simulink model "PEM_cell_validate_static"  (R2025b)
settings: Solver=ode23t  StartTime=0.0  StopTime=6895  RelTol=1e-3
values from neighbouring files (symbols this model uses):
  Active_Area = 17.64    [PV_PEM_direct_battery_active.m]    (also in PV_PEM_direct_battery_passive.m; PV_PEM_indirect_battery.m; PV_PEM_reconfigurable_battery.m; Sim_vs_meas_dynamic.m)
  Input_Time = T{:,5}    [Sim_vs_meas_dynamic.m]
  Input_Voltage = T{:,16}    [Sim_vs_meas_dynamic.m]
  Ra = 0.00177    [PV_PEM_direct_battery_active.m]    (also in PV_PEM_direct_battery_passive.m; PV_PEM_indirect_battery.m; PV_PEM_reconfigurable_battery.m; Sim_vs_meas_dynamic.m)
  Rc = 0.0005    [PV_PEM_direct_battery_active.m]    (also in PV_PEM_direct_battery_passive.m; PV_PEM_indirect_battery.m; PV_PEM_reconfigurable_battery.m; Sim_vs_meas_dynamic.m)
  Rint = 0.008673    [PV_PEM_direct_battery_active.m]    (also in PV_PEM_direct_battery_passive.m; PV_PEM_indirect_battery.m; PV_PEM_reconfigurable_battery.m; Sim_vs_meas_dynamic.m)
  Vint = 1.475841    [PV_PEM_direct_battery_active.m]    (also in PV_PEM_direct_battery_passive.m; PV_PEM_indirect_battery.m; PV_PEM_reconfigurable_battery.m; Sim_vs_meas_dynamic.m)
libraries: fl_lib x15, nesl_utility x9, simulink x6
settings Model: Creator=hanna  LastModifiedBy=hanna
settings DataIOCC: SignalLogging=off  StreamToWks=off  ReturnWorkspaceOutputs=off
settings DebuggingCC: SaveWithParameterizedLinksMsg=none

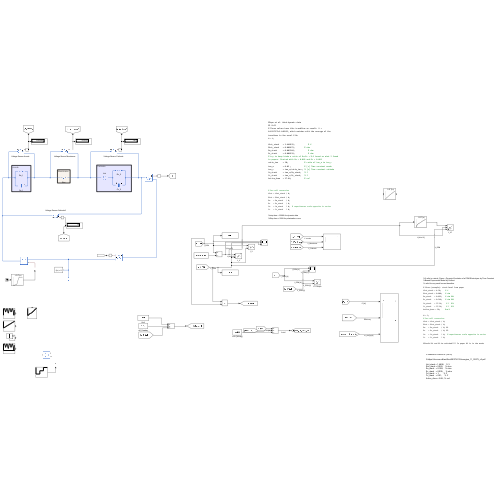
[thumbnail: Simulink's stored preview of the top-level diagram]
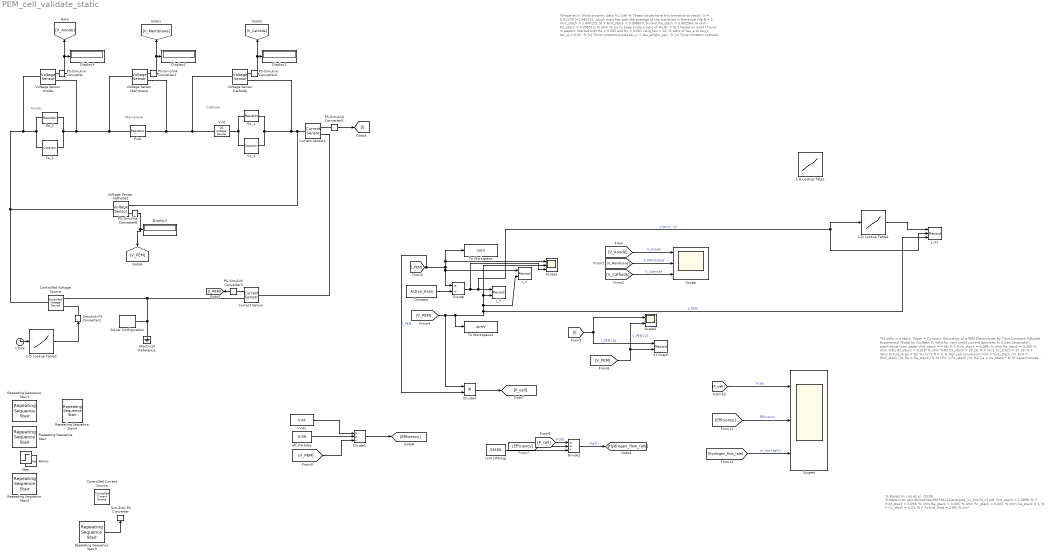
== system PEM_cell_validate_static ==
  note: %Pape et al. Wind dynamic data
      | %1 Cell
      | % These values have this trendline as result: V = 0.01175*I+1.440125, which matches with the average of the trendines in the excel file
      | N = 1;
      |
      | Vint_stack = 1.440155; % V
      | Rint_stack = 0.008673; % ohm
      | Ra_stack = 0.002564; % ohm
      | Rc_stack = 0.000513; % ohm
      | % try to keep kinda a ratio of Ra:Rc = %:1 based on what I found in papers. Started with Ra = 0.005 and Rc = 0.001
      | ratio_tau = 10; % ratio of tau_a to tau_c
      | tau_a = 0.05 ; % [s] Time constant anode
      | tau_c = tau_a/ratio_tau ; % [s] Time constant cathode
      | Ca_stack = tau_a/Ra_stack; % F
      | Cc_stack = tau_c/Rc_stack; % F
      | Active_Area = 17.64; % cm²
      |
      | % Per-cell conversion
      | Vint = Vint_stack / N;
      | Rint = Rint_stack / N;
      | Ra = Ra_stack / N;
      | Rc = Rc_stack / N;
      | Ca = Ca_stack * N; % capacitances scale opposite in series
      | Cc = Cc_stack * N;
      |
      | %stop time = 29988 for dynamic data
      | %Stop time = 5099 for polarisation curve
  note: % Based on Liso et al. (2018)
      | %https://vbn.aau.dk/ws/files/293736112/energies_11_03273_v2.pdf
      | Vint_stack = 1.4898; % V
      | Rint_stack = 0.093; % ohm
      | Ra_stack = 0.005; % ohm
      | Rc_stack = 0.005; % ohm
      | Ca_stack = 1; % F
      | Cc_stack = 0.01; % F
      | Active_Area = 2.89; % cm²
  note: %3 cells in a stack: Paper = Dynamic Emulation of a PEM Electrolyzer by Time Constant %Based Exponential Model by Guilbert
      | % valid for very small current densities
      |
      | % Given (example): stack-level from paper
      | Vint_stack = 4.38; % V
      | Rint_stack = 0.088; % ohm
      | Ra_stack = 0.035; % ohm %R1
      | Rc_stack = 0.318; % ohm %R2
      | Ca_stack = 37.26; % F %C1
      | Cc_stack = 37.26; % F %C2
      | Active_Area = 50; %cm^2
      |
      | N = 3;
      | % Per-cell conversion
      | Vint = Vint_stack / N;
      | Rint = Rint_stack / N;
      | Ra = Ra_stack / N; %1
      | Rc = Rc_stack / N; %2
      | Ca = Ca_stack * N; % capacitances scale opposite in series
      | Cc = Cc_stack * N;
      |
      | %Should R1 and R2 be switched???? In paper R2 is in the anode
  note: Cathode
  note: Anode
  note: Membrane
  1-D Lookup Table : Lookup_n-D  NumberOfTableDimensions=1  BreakpointsForDimension1=|  Table=|  InternalRulePriority=Speed  RndMeth=Simplest
      BreakpointsForDimension1=|
      | [0.0385
      | 0.0963
      | 0.1784
      | 0.3065
      | 0.4043
      | 0.6017
      | 0.8000
      | 0.9971
      | 1.1935
      | 1.3913
      | 1.5897
      | 1.7870
      | 1.9839 ]
      Table=|
      | [1.4682
      | 1.5069
      | 1.5423
      | 1.5870
      | 1.6183
      | 1.6780
      | 1.7357
      | 1.7924
      | 1.8478
      | 1.8992
      | 1.9511
      | 1.9983
      | 2.0476 ]
  1-D Lookup Table1 : Lookup_n-D  NumberOfTableDimensions=1  BreakpointsForDimension1=[0.002196, 0.005037, 0.010062, 0.020117, 0.030138, 0.040142, 0.060187, 0.080224, 0.100238, 0.150326, 0.200385, 0.250495, 0.297237, 0.347374, 0.397259, 0.447324, 0.497136, 0.597415, 0.697348, 0.79707, 0.99733, 1.097498, 1.197311, 1.297265, 1.397199, 1.497192, 1.597162, 1.696959, 1.79709, 1.896997, 1.997028]  Table=[1.320659, 1.36234, 1.375311, 1.392194, 1.403544, 1.412891, 1.429582, 1.444366, 1.456766, 1.485284, 1.509416, 1.531258, 1.548522, 1.565118, 1.580856, 1.596021, 1.60947, 1.636368, 1.660976, 1.686156, 1.734229, 1.758361, 1.782015, 1.806052, 1.829134, 1.853552, 1.875967, 1.899622, 1.924231, 1.948363, 1.971923]  InternalRulePriority=Speed  RndMeth=Simplest
  1-D Lookup Table2 : Lookup_n-D  NumberOfTableDimensions=1  BreakpointsForDimension1=Input_Time  Table=Input_Voltage  InternalRulePriority=Speed  RndMeth=Simplest
  Ca_1 : fl_lib/Electrical/Electrical Elements/Capacitor  c=Ca F  r=1e-6 Ohm  g=0 1/Ohm  i_specify=off  i_priority=None  i=0 A  i_nominal_specify=off  i_nominal_value=1  i_nominal_unit=A  v_specify=off  v_priority=None  v=0 V  v_nominal_specify=off  v_nominal_value=1  v_nominal_unit=V  vc_specify=off  vc_priority=High  vc=0 V  vc_nominal_specify=off  vc_nominal_value=1  vc_nominal_unit=V
  Cc_2 : fl_lib/Electrical/Electrical Elements/Capacitor  c=Cc F  r=1e-6 Ohm  g=0 1/Ohm  i_specify=off  i_priority=None  i=0 A  i_nominal_specify=off  i_nominal_value=1  i_nominal_unit=A  v_specify=off  v_priority=None  v=0 V  v_nominal_specify=off  v_nominal_value=1  v_nominal_unit=V  vc_specify=off  vc_priority=High  vc=0 V  vc_nominal_specify=off  vc_nominal_value=1  vc_nominal_unit=V
  Clock : Clock
  Constant : Constant  Value=Active_Area
  Controlled Current Source : fl_lib/Electrical/Electrical Sources/Controlled Current Source
  Controlled Voltage Source : fl_lib/Electrical/Electrical Sources/Controlled Voltage Source
  Current Sensor : fl_lib/Electrical/Electrical Sensors/Current Sensor
  Current Sensor1 : fl_lib/Electrical/Electrical Sensors/Current Sensor
  Display{1..4} (4 alike) : Display
  Divide : Product  Inputs=*/
  Divide1 : Product  Inputs=**/
  Divide2 : Product  Inputs=**/
  Divide4 : Product  Inputs=**
  Electrical Reference : fl_lib/Electrical/Electrical Elements/Electrical Reference
  I_V : Record  NumPorts=2.0  FileSettingsInternal="{\"entries\":[{\"content\":{\"excelSettings\":{\"content\":{},\"type\":\"Streamout.ExcelSettings\"},\"parquetSettings\":{\"content\":{},\"type\":\"Streamout.ParquetSettings\"}},\"type\":\"Streamout.FileSettingStorage\",\"uuid\":\"\"}],\"packageUris\":[\"http:\\/\\/schema.mathworks.com\\/mf0\\/streamout_blocks\\/R2020a\"],\"version\":\"1.0\"}"  FrameSettings=[0, 0]  Layout=[1 1]  SignalsInternal="{\"entries\":[{\"content\":{\"signals\":[{\"content\":{\"blockPath\":[],\"dimensions\":[1],\"domain\":\"\",\"lineColor\":\"#ff6929\",\"lineWidth\":2,\"plots\":[ 1 ],\"port\":1,\"sid\":[\"\"],\"signalID\":1,\"signalName\":\"I_PEM\"},\"type\":\"RecordBlkView.Signal\",\"uuid\":\"\"},{\"content\":{\"blockPath\":[],\"dimensions\":[1],\"domain\":\"\",\"lineColor\":\"#64d413\",\"lineWidth\":2,\"plots\":[ 1 ],\"port\":2,\"sid\":[\"\"],\"signalID\":2,\"signalName\":\"V_PEM\"},\"type\":\"RecordBlkView.Signal\",\"uuid\":\"\"}]},\"type\":\"RecordBlkView.InputSignals\",\"uuid\":\"\"}],\"packageUris\":[\"http:\\/\\/schema.mathworks.com\\/mf0\\/streamout_blocks\\/R2020a\"],\"version\":\"1.0\"}"  VisualizationBindings="{\"xyplotplugin\":{\"info\":[{\"series\":[{\"bindingParametersList\":[{\"parameter\":\"X-Axis\",\"signalID\":1,\"signalName\":\"I_PEM\"},{\"parameter\":\"Y-Axis\",\"signalID\":2,\"signalName\":\"V_PEM\"}],\"seriesID\":0}],\"subplotID\":1}]}}"  CompatibilityTag=XY
  J_V : Record  NumPorts=2.0  FileSettingsInternal="{\"entries\":[{\"content\":{\"excelSettings\":{\"content\":{},\"type\":\"Streamout.ExcelSettings\"},\"parquetSettings\":{\"content\":{},\"type\":\"Streamout.ParquetSettings\"}},\"type\":\"Streamout.FileSettingStorage\",\"uuid\":\"\"}],\"packageUris\":[\"http:\\/\\/schema.mathworks.com\\/mf0\\/streamout_blocks\\/R2020a\"],\"version\":\"1.0\"}"  FrameSettings=[0, 0]  Layout=[1 1]  SignalsInternal="{\"entries\":[{\"content\":{\"signals\":[{\"content\":{\"blockPath\":[],\"dimensions\":[1],\"domain\":\"\",\"lineColor\":\"#a2142f\",\"plots\":[ 1 ],\"port\":1,\"sid\":[\"\"],\"signalID\":1,\"signalName\":\"J [A\\/cm^2]\"},\"type\":\"RecordBlkView.Signal\",\"uuid\":\"\"},{\"content\":{\"blockPath\":[],\"dimensions\":[1],\"domain\":\"\",\"lineColor\":\"#139fff\",\"plots\":[ 1 ],\"port\":2,\"sid\":[\"\"],\"signalID\":2,\"signalName\":\"V_PEM\"},\"type\":\"RecordBlkView.Signal\",\"uuid\":\"\"}]},\"type\":\"RecordBlkView.InputSignals\",\"uuid\":\"\"}],\"packageUris\":[\"http:\\/\\/schema.mathworks.com\\/mf0\\/streamout_blocks\\/R2020a\"],\"version\":\"1.0\"}"  VisualizationBindings="{\"xyplotplugin\":{\"info\":[{\"series\":[{\"bindingParametersList\":[{\"parameter\":\"X-Axis\",\"signalID\":1,\"signalName\":\"J [A\\/cm^2]\"},{\"parameter\":\"Y-Axis\",\"signalID\":2,\"signalName\":\"V_PEM\"}],\"seriesID\":0}],\"subplotID\":1}]}}"  CompatibilityTag=XY
  J_V1 : Record  NumPorts=3.0  FileSettingsInternal="{\"entries\":[{\"content\":{\"excelSettings\":{\"content\":{},\"type\":\"Streamout.ExcelSettings\"},\"parquetSettings\":{\"content\":{},\"type\":\"Streamout.ParquetSettings\"}},\"type\":\"Streamout.FileSettingStorage\",\"uuid\":\"\"}],\"packageUris\":[\"http:\\/\\/schema.mathworks.com\\/mf0\\/streamout_blocks\\/R2020a\"],\"version\":\"1.0\"}"  FrameSettings=[0, 0, 0]  Layout=[1 1]  SignalsInternal="{\"entries\":[{\"content\":{\"signals\":[{\"content\":{\"blockPath\":[],\"dimensions\":[1],\"domain\":\"\",\"lineColor\":\"#64d413\",\"lineWidth\":2,\"plots\":[ 1 ],\"port\":1,\"sid\":[\"\"],\"signalID\":1,\"signalName\":\"1-D Lookup\\nTable1\"},\"type\":\"RecordBlkView.Signal\",\"uuid\":\"\"},{\"content\":{\"blockPath\":[],\"dimensions\":[1],\"domain\":\"\",\"lineColor\":\"#ff13a6\",\"lineWidth\":2,\"plots\":[ 1 ],\"port\":2,\"sid\":[\"\"],\"signalID\":2,\"signalName\":\"J [A\\/cm^2]\"},\"type\":\"RecordBlkView.Signal\",\"uuid\":\"\"},{\"content\":{\"blockPath\":[],\"dimensions\":[1],\"domain\":\"\",\"lineColor\":\"#fe330a\",\"lineWidth\":2,\"plots\":[ 1 ],\"port\":3,\"sid\":[\"\"],\"signalID\":3,\"signalName\":\"V_PEM\"},\"type\":\"RecordBlkView.Signal\",\"uuid\":\"\"}]},\"type\":\"RecordBlkView.InputSignals\",\"uuid\":\"\"}],\"packageUris\":[\"http:\\/\\/schema.mathworks.com\\/mf0\\/streamout_blocks\\/R2020a\"],\"version\":\"1.0\"}"  VisualizationBindings="{\"xyplotplugin\":{\"info\":[{\"series\":[{\"bindingParametersList\":[{\"parameter\":\"X-Axis\",\"signalID\":2,\"signalName\":\"J [A\\/cm^2]\"},{\"parameter\":\"Y-Axis\",\"signalID\":1,\"signalName\":\"1-D Lookup\\nTable1\"}],\"seriesID\":0},{\"bindingParametersList\":[{\"parameter\":\"X-Axis\",\"signalID\":2,\"signalName\":\"J [A\\/cm^2]\"},{\"parameter\":\"Y-Axis\",\"signalID\":3,\"signalName\":\"V_PEM\"}],\"seriesID\":1}],\"subplotID\":1}]}}"  CompatibilityTag=XY
  LHV [Wh/kg] : Constant  Value=33400
  PS-Simulink Converter{,1..3,5..6} (6 alike) : nesl_utility/PS-Simulink Converter  PhysicalDomain=network_engine_domain  SubClassName=ps_output  LeftPortType=input  RightPortType=output  PseudoPeriodic=off  Frequencies=[]  VectorFormat=inherit  Unit=inherit  AffineConversion=off
  Ra_1 : fl_lib/Electrical/Electrical Elements/Resistor  R=Ra Ohm  i_specify=off  i_priority=None  i=0 A  i_nominal_specify=off  i_nominal_value=1  i_nominal_unit=A  v_specify=off  v_priority=None  v=0 V  v_nominal_specify=off  v_nominal_value=1  v_nominal_unit=V
  Ramp : simulink/Sources/Ramp  slope=0.02  start=0  InitialOutput=0
  Rc_2 : fl_lib/Electrical/Electrical Elements/Resistor  R=Rc Ohm  i_specify=off  i_priority=None  i=0 A  i_nominal_specify=off  i_nominal_value=1  i_nominal_unit=A  v_specify=off  v_priority=None  v=0 V  v_nominal_specify=off  v_nominal_value=1  v_nominal_unit=V
  Repeating Sequence Stair : simulink/Sources/Repeating Sequence Stair  OutValues=[2:2:50]  tsamp=50  OutMin=[]  OutMax=[]  OutDataTypeStr=double  OutputDataTypeScalingMode=double  OutDataType=fixdt(0,8)  ConRadixGroup=Best Precision: Vector-wise  OutScaling=2^-12
  Repeating Sequence Stair1 : simulink/Sources/Repeating Sequence Stair  OutValues=[40.000, 41.843, 43.685, 45.524, 47.360, 49.191, 50.000, 50.000, 50.000, 50.000, 50.000, 50.000, 50.000, 50.000, 50.000, 50.000, 50.000, 50.000, 50.000, 50.000, 50.000, 50.000, 49.310, 47.829, 46.329, 44.809, 43.269, 41.709, 40.129, 38.530, 36.911, 35.274, 33.618, 31.944, 30.253, 28.545, 26.821, 25.082, 25.429, 26.717, 27.993, 29.257, 30.511, 31.756, 32.992, 34.221, 35.444, 36.663, 37.878, 39.091, 40.303, 41.515, 42.729, 43.946, 45.167, 46.393, 47.625, 48.865, 50.000, 50.000, 50.000, 50.000, 50.000, 50.000, 50.000, 50.000, 48.899, 47.217, 45.552, 43.905, 42.277, 40.668, 39.079, 37.509, 35.959, 34.429, 32.918, 31.428, 29.957, 28.506, 27.074, 25.661, 24.266, 22.889, 21.529, 20.186, 18.859, 17.546, 19.112, 20.882, 22.665, 24.458, 26.262, 28.075, 29.896, 31.724, 33.557, 35.395, 37.236, 39.078, 40.922, 42.764, 44.605, 46.443, 48.276, 50.000, 50.000, 50.000, 50.000, 50.000, 50.000, 50.000, 50.000, 50.000, 50.000, 50.000, 50.000, 50.000, 50.000, 50.000, 50.000, 50.000, 48.572, 47.082, 45.571, 44.041, 42.491, 40.921, 39.332, 37.723, 36.095, 34.448, 32.783, 31.101, 29.401, 27.685, 25.953, 24.780, 26.075, 27.357, 28.627, 29.886, 31.135, 32.375, 33.607, 34.833, 36.054, 37.271, 38.485, 39.697, 40.909, 42.122, 43.337, 44.556, 45.779, 47.008, 48.244, 49.489, 50.000, 50.000, 50.000, 50.000, 50.000, 50.000, 50.000, 49.747, 48.056, 46.382, 44.726, 43.089, 41.470, 39.871, 38.291, 36.731, 35.191, 33.671, 32.171, 30.690, 29.229, 27.788, 26.365, 24.961, 23.575, 22.207, 20.856, 19.520, 18.200, 18.232,10, 5,1, 19.995, 21.772, 23.560, 25.359, 27.168, 28.985, 30.809, 32.640, 34.476, 36.315, 38.157, 40.000]  tsamp=1  OutMin=[]  OutMax=[]  OutDataTypeStr=double  OutputDataTypeScalingMode=double  OutDataType=fixdt(0,8)  ConRadixGroup=Best Precision: Vector-wise  OutScaling=2^-12
  Repeating Sequence Stair2 : simulink/Sources/Repeating Sequence Stair  OutValues=[1.751, 1.834, 1.917, 1.999, 2.082, 2.164, 2.200, 2.200, 2.200, 2.200, 2.200, 2.200, 2.200, 2.200, 2.200, 2.200, 2.200, 2.200, 2.200, 2.200, 2.200, 2.200, 2.169, 2.103, 2.036, 1.967, 1.898, 1.828, 1.757, 1.685, 1.613, 1.540, 1.465, 1.390, 1.314, 1.238, 1.160, 1.082, 1.097, 1.154, 1.211, 1.268, 1.324, 1.380, 1.436, 1.491, 1.546, 1.601, 1.656, 1.710, 1.764, 1.819, 1.873, 1.927, 1.982, 2.037, 2.093, 2.148, 2.200, 2.200, 2.200, 2.200, 2.200, 2.200, 2.200, 2.200, 2.151, 2.076, 2.002, 1.928, 1.855, 1.783, 1.712, 1.641, 1.572, 1.503, 1.435, 1.368, 1.302, 1.237, 1.173, 1.110, 1.048, 0.987, 0.927, 0.869, 0.811, 0.754, 0.823, 0.903, 0.983, 1.064, 1.145, 1.226, 1.308, 1.390, 1.473, 1.555, 1.638, 1.720, 1.803, 1.885, 1.968, 2.050, 2.132, 2.200, 2.200, 2.200, 2.200, 2.200, 2.200, 2.200, 2.200, 2.200, 2.200, 2.200, 2.200, 2.200, 2.200, 2.200, 2.200, 2.200, 2.136, 2.069, 2.001, 1.932, 1.863, 1.793, 1.721, 1.650, 1.577, 1.503, 1.428, 1.352, 1.276, 1.199, 1.121, 1.068, 1.126, 1.183, 1.240, 1.296, 1.352, 1.408, 1.463, 1.518, 1.573, 1.628, 1.682, 1.737, 1.791, 1.845, 1.900, 1.955, 2.010, 2.065, 2.121, 2.176, 2.200, 2.200, 2.200, 2.200, 2.200, 2.200, 2.200, 2.189, 2.114, 2.039, 1.965, 1.892, 1.819, 1.748, 1.677, 1.607, 1.538, 1.470, 1.403, 1.337, 1.272, 1.208, 1.145, 1.083, 1.022, 0.961, 0.902, 0.843, 0.785, 0.787, 0.404, 0.180, 0.000, 0.808, 0.887, 0.967, 1.047, 1.128, 1.209, 1.290, 1.372, 1.454, 1.536, 1.619, 1.702, 1.751]  tsamp=1  OutMin=[]  OutMax=[]  OutDataTypeStr=double  OutputDataTypeScalingMode=double  OutDataType=fixdt(0,8)  ConRadixGroup=Best Precision: Vector-wise  OutScaling=2^-12
  Repeating Sequence Stair3 : simulink/Sources/Repeating Sequence Stair  OutValues=[10,30,50]  tsamp=50  OutMin=[]  OutMax=[]  OutDataTypeStr=double  OutputDataTypeScalingMode=double  OutDataType=fixdt(0,8)  ConRadixGroup=Best Precision: Vector-wise  OutScaling=2^-12
  Repeating Sequence Stair4 : simulink/Sources/Repeating Sequence Stair  OutValues=[1.3, 1.35, 1.4, 1.45, 1.48, 1.5 1.53, 1.55, 1.6, 1.65, 1.7, 1.75, 1.8, 1.85, 1.9, 1.95, 2.0]  tsamp=300  OutMin=[]  OutMax=[]  OutDataTypeStr=double  OutputDataTypeScalingMode=double  OutDataType=fixdt(0,8)  ConRadixGroup=Best Precision: Vector-wise  OutScaling=2^-12
  Rint : fl_lib/Electrical/Electrical Elements/Resistor  R=Rint Ohm  i_specify=off  i_priority=None  i=0 A  i_nominal_specify=off  i_nominal_value=1  i_nominal_unit=A  v_specify=off  v_priority=None  v=0 V  v_nominal_specify=off  v_nominal_value=1  v_nominal_unit=V
  Scope : Scope  NumInputPorts=3
      settings: ActiveDisplayYMinimum=-0.025574999999999994  ActiveDisplayYMaximum=0.23017500000000002  DataLoggingVariableName=ScopeData3
  Scope1 : Scope  NumInputPorts=3
      settings: ActiveDisplayYMinimum=2.1952046709351865  ActiveDisplayYMaximum=2.2345014292442293  DataLoggingVariableName=ScopeData2
  Scope2 : Scope  NumInputPorts=2
      settings: ActiveDisplayYMinimum=-5.9214977117401686  ActiveDisplayYMaximum=31.360438509949088  DataLoggingVariableName=ScopeData4
  Scope4 : Scope  NumInputPorts=3
      settings: ActiveDisplayString=3  ActiveDisplayYMinimum=-0.00015500111670992237  ActiveDisplayYMaximum=0.0023420023487162834
  Simulink-PS Converter : nesl_utility/Simulink-PS Converter  PhysicalDomain=network_engine_domain  SubClassName=ps_input  LeftPortType=input  RightPortType=output  PseudoPeriodic=off  Frequencies=[]  NoiseDistribution=none  NoiseParameters=[]  Unit=1  AffineConversion=off  FilteringAndDerivatives=provide  SimscapeFilterOrder=1  InputFilterTimeConstant=0.001  UdotUserProvided=0
  Simulink-PS Converter1 : nesl_utility/Simulink-PS Converter  PhysicalDomain=network_engine_domain  SubClassName=ps_input  LeftPortType=input  RightPortType=output  PseudoPeriodic=off  Frequencies=[]  NoiseDistribution=none  NoiseParameters=[]  Unit=1  AffineConversion=off  FilteringAndDerivatives=provide  SimscapeFilterOrder=1  InputFilterTimeConstant=0.001  UdotUserProvided=0
  Solver Configuration : nesl_utility/Solver Configuration  PhysicalDomain=network_engine_domain  SubClassName=solver  LeftPortType=input  RightPortType=generic  Tones=[]  Harmonics=[]  SimulateNoise=off  Profile=off  UseLocalSampling=off  EnableSwitchedLinearOptims=on  FrequencyDomain=off  UseCCode=off  RelTol=0.001  AbsTol=0.001  MinStep=1e-09  ToWorkspace=off  RevertToSquareIcSolve=off  NumHomotopyIterations=100  PhasorMode=off  PhasorModeNumHarmonics=1  ConsistencySolver=NEWTON_XTOL_AFTER_FTOL  IndexReductionMethod=DerivativeReplacement  DoDC=off  ResidualTolerance=1e-09  ConsistencyTolSource=GLOBAL  ConsistencyAbsTol=0.001  ConsistencyRelTol=0.001  ConsistencyTolFactor=0.001  UseLocalSolver=off  LocalSolverChoice=NE_BACKWARD_EULER_ADVANCER  ResolveIndetEquations=on  FunctionEvalNumThread=1  LocalSolverSampleTime=0.001  DoFixedCost=off  MaxNonlinIter=3  MaxModeIter=2  ComputeImpulses=off  ImpulseIterations=2  LinearAlgebra=auto  LinearAlgebraNumThread=0  EquationFormulation=NE_TIME_EF  DelaysMemoryBudget=1024  AutomaticFiltering=on  FilteringTimeConstant=0.001  PartitionStorageMethod=AS_NEEDED  PartitionMemoryBudget=1024  PartitionMethod=ROBUST  MultibodyUseLocalSolver=off  MultibodyLocalSolverChoice=ODE1  MultibodyLocalSolverSampleTime=0.001
  Step : Step  Time=100  Before=5.45  After=6.25  SampleTime=0
  To Workspace : ToWorkspace  VariableName=simI  SaveFormat=Timeseries  SampleTime=0.1
  To Workspace1 : ToWorkspace  VariableName=simV  SaveFormat=Timeseries  SampleTime=0.1
  Vint : fl_lib/Electrical/Electrical Sources/DC Voltage Source  v0=Vint V
  Vint1 : Constant  Value=Vint
  Voltage Sensor Anode : fl_lib/Electrical/Electrical Sensors/Voltage Sensor
  Voltage Sensor Cathode : fl_lib/Electrical/Electrical Sensors/Voltage Sensor
  Voltage Sensor Cathode2 : fl_lib/Electrical/Electrical Sensors/Voltage Sensor
  Voltage Sensor Membrane : fl_lib/Electrical/Electrical Sensors/Voltage Sensor
  XY Graph : Record  NumPorts=2.0  FileSettingsInternal="{\"entries\":[{\"content\":{\"excelSettings\":{\"content\":{},\"type\":\"Streamout.ExcelSettings\"},\"parquetSettings\":{\"content\":{},\"type\":\"Streamout.ParquetSettings\"}},\"type\":\"Streamout.FileSettingStorage\",\"uuid\":\"\"}],\"packageUris\":[\"http:\\/\\/schema.mathworks.com\\/mf0\\/streamout_blocks\\/R2020a\"],\"version\":\"1.0\"}"  FrameSettings=[0, 0]  Layout=[1 1]  SignalsInternal="{\"entries\":[{\"content\":{\"signals\":[{\"content\":{\"blockPath\":[],\"dimensions\":[1],\"domain\":\"\",\"lineColor\":\"#a2142f\",\"lineWidth\":2,\"plots\":[ 1 ],\"port\":1,\"sid\":[\"\"],\"signalID\":1,\"signalName\":\"I_PEM [A]\"},\"type\":\"RecordBlkView.Signal\",\"uuid\":\"\"},{\"content\":{\"blockPath\":[],\"dimensions\":[1],\"domain\":\"\",\"lineColor\":\"#139fff\",\"lineWidth\":2,\"plots\":[ 1 ],\"port\":2,\"sid\":[\"\"],\"signalID\":2,\"signalName\":\"V_PEM [V]\"},\"type\":\"RecordBlkView.Signal\",\"uuid\":\"\"}]},\"type\":\"RecordBlkView.InputSignals\",\"uuid\":\"\"}],\"packageUris\":[\"http:\\/\\/schema.mathworks.com\\/mf0\\/streamout_blocks\\/R2020a\"],\"version\":\"1.0\"}"  VisualizationBindings="{\"xyplotplugin\":{\"info\":[{\"series\":[{\"bindingParametersList\":[{\"parameter\":\"X-Axis\",\"signalID\":1,\"signalName\":\"I_PEM [A]\"},{\"parameter\":\"Y-Axis\",\"signalID\":2,\"signalName\":\"V_PEM [V]\"}],\"seriesID\":0}],\"subplotID\":1}]}}"  CompatibilityTag=XY
  eff_Faraday : Constant  Value=0.99
  wires:
  [V_PEM] -> Divide4/1, To Workspace1/1, J_V1/3, Scope1/2, J_V/2, I_V/2  "V_PEM"
  PS-Simulink Converter3/1 -> [I_PEM]
  [I_PEM] -> Scope1/1, To Workspace/1, Divide/1, I_V/1, Divide4/2  "I_PEM"
  Divide/1 -> Scope1/3, 1-D Lookup Table1/1, J_V1/2, J_V/1  "J [A/cm^2]"
  Constant/1 -> Divide/2
  [V_Anode] -> Scope/1  "V_anode"
  PS-Simulink Converter6/1 -> [V_PEM], Display3/1
  [V_Membrane] -> Scope/2  "V_Membrane"
  PS-Simulink Converter5/1 -> [I]
  PS-Simulink Converter/1 -> [V_Anode], Display4/1
  PS-Simulink Converter1/1 -> [V_Membrane], Display1/1
  [V_PEM] -> Scope2/2, XY Graph/2  "V_PEM [V]"
  [V_Cathode] -> Scope/3  "V_Cathode"
  [I] -> Scope2/1, XY Graph/1  "I_PEM [A]"
  PS-Simulink Converter2/1 -> [V_Cathode], Display2/1
  Divide4/1 -> [P_cell]
  [P_cell] -> Divide1/1  "P [W]"
  LHV [Wh/kg]/1 -> Divide1/3
  Divide1/1 -> [Hydrogen_flow_rate]  "[kg/h]"
  [Efficiency] -> Divide1/2
  [V_PEM] -> Divide2/3
  Vint1/1 -> Divide2/1
  eff_Faraday/1 -> Divide2/2
  Divide2/1 -> [Efficiency]
  [Hydrogen_flow_rate] -> Scope4/3  "m_dot [kg/h]"
  [Efficiency] -> Scope4/2  "Efficiency"
  [P_cell] -> Scope4/1  "P [W]"
  1-D Lookup Table1/1 -> J_V1/1
  Clock/1 -> 1-D Lookup Table2/1
  Repeating Sequence Stair3/1 -> Simulink-PS Converter/1
  1-D Lookup Table2/1 -> Simulink-PS Converter1/1
  connections:
  Electrical Reference/LConn1 -- Controlled Voltage Source/RConn2 -- Current Sensor/RConn2 -- Solver Configuration/RConn1
  PS-Simulink Converter3/LConn1 -- Current Sensor/RConn1
  Ca_1/RConn1 -- Ra_1/RConn1 -- Voltage Sensor Anode/RConn2 -- Voltage Sensor Membrane/LConn1 -- Rint/LConn1
  Current Sensor1/LConn1 -- Rc_2/RConn1 -- Cc_2/RConn1 -- Voltage Sensor Cathode/RConn2 -- Voltage Sensor Cathode2/RConn2
  Vint/LConn1 -- Rint/RConn1 -- Voltage Sensor Membrane/RConn2 -- Voltage Sensor Cathode/LConn1
  Cc_2/LConn1 -- Rc_2/LConn1 -- Vint/RConn1
  Voltage Sensor Cathode2/LConn1 -- Controlled Voltage Source/LConn1 -- Voltage Sensor Anode/LConn1 -- Ra_1/LConn1 -- Ca_1/LConn1
  Voltage Sensor Cathode2/RConn1 -- PS-Simulink Converter6/LConn1
  Voltage Sensor Cathode/RConn1 -- PS-Simulink Converter2/LConn1
  PS-Simulink Converter5/LConn1 -- Current Sensor1/RConn1
  Current Sensor1/RConn2 -- Current Sensor/LConn1
  Voltage Sensor Membrane/RConn1 -- PS-Simulink Converter1/LConn1
  Voltage Sensor Anode/RConn1 -- PS-Simulink Converter/LConn1
  Simulink-PS Converter1/RConn1 -- Controlled Voltage Source/RConn1
